simulink model "Lab1_419_simul3"  (R2023b)
settings: Solver=VariableStepAuto  StartTime=0.0  StopTime=120  RelTol=1e-9
settings Model: Creator=Aiden  LastModifiedBy=julia

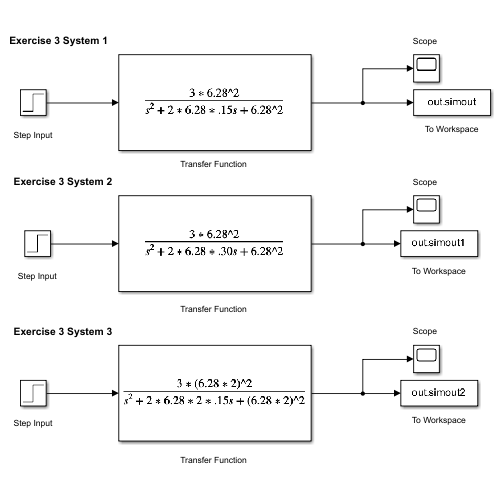
[thumbnail: Simulink's stored preview of the top-level diagram]
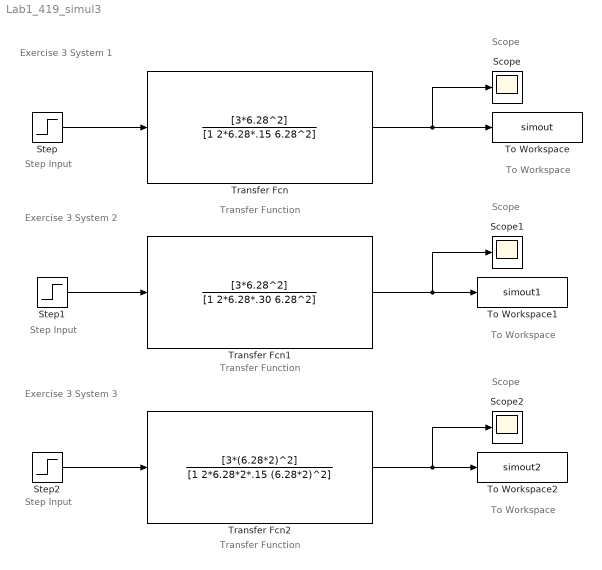
== system Lab1_419_simul3 ==
  note: Step Input
  note: Scope
  note: To Workspace
  note: Transfer Function
  note: Exercise 3 System 1
  note: Exercise 3 System 2
  note: Exercise 3 System 3
  note: Transfer Function
  note: Transfer Function
  note: To Workspace
  note: To Workspace
  note: Scope
  note: Scope
  note: Step Input
  note: Step Input
  Scope : Scope
  Scope1 : Scope
  Scope2 : Scope
  Step : Step  SampleTime=0
  Step1 : Step  SampleTime=0
  Step2 : Step  SampleTime=0
  To Workspace : ToWorkspace  VariableName=simout  SampleTime=-1
  To Workspace1 : ToWorkspace  VariableName=simout1  SampleTime=-1
  To Workspace2 : ToWorkspace  VariableName=simout2  SampleTime=-1
  Transfer Fcn : TransferFcn  Numerator=[3*6.28^2]  Denominator=[1 2*6.28*.15 6.28^2]
  Transfer Fcn1 : TransferFcn  Numerator=[3*6.28^2]  Denominator=[1 2*6.28*.30 6.28^2]
  Transfer Fcn2 : TransferFcn  Numerator=[3*(6.28*2)^2]  Denominator=[1 2*6.28*2*.15 (6.28*2)^2]
  wires:
  Step/1 -> Transfer Fcn/1
  Transfer Fcn/1 -> To Workspace/1, Scope/1
  Step1/1 -> Transfer Fcn1/1
  Transfer Fcn1/1 -> To Workspace1/1, Scope1/1
  Transfer Fcn2/1 -> Scope2/1, To Workspace2/1
  Step2/1 -> Transfer Fcn2/1
